simulink model "control"  (R2020b)
settings: Solver=VariableStepAuto  StartTime=0.0  StopTime=10.0  RelTol=1e-3
settings Model: Creator=Varun  LastModifiedBy=Varun
settings DataIOCC: SaveOutput=off  SaveTime=off

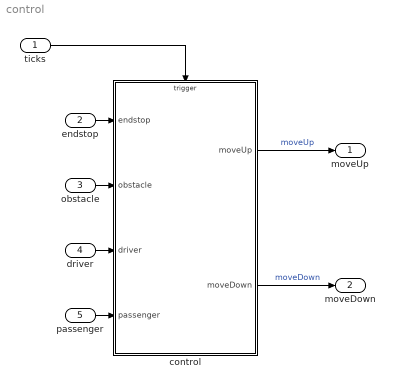
== system control ==
  ticks : Inport  OutDataTypeStr=double  PortDimensions=1
  endstop : Inport  Port=2  OutDataTypeStr=boolean  PortDimensions=1
  obstacle : Inport  Port=3  OutDataTypeStr=boolean  PortDimensions=1
  driver : Inport  Port=4  OutDataTypeStr=boolean  PortDimensions=3
  passenger : Inport  Port=5  OutDataTypeStr=boolean  PortDimensions=3
  control : Stateflow chart  TreatAsAtomicUnit=on
  moveUp : Outport  OutDataTypeStr=boolean  PortDimensions=1
  moveDown : Outport  Port=2  OutDataTypeStr=boolean  PortDimensions=1
  wires:
  passenger/1 -> control/4(passenger)
  obstacle/1 -> control/2(obstacle)
  control/2(moveDown) -> moveDown/1  "moveDown"
  ticks/1 -> control/Trigger
  control/1(moveUp) -> moveUp/1  "moveUp"
  endstop/1 -> control/1(endstop)
  driver/1 -> control/3(driver)

== stateflow chart control/control ==
  settings: executeAtInitialization=1
  state safe
    state driverNeutral
      entry:
      moveUp = 0;
      moveDown = 0;
      state passengerneutral
        entry:
        moveUp = 0;
        moveDown = 0;
      state passengerDown
        entry: moveDown = 1;
        exit: moveDown = 0;
        state iniPassengerDown
        state passengerDown
        state autoPassengerDown
        iniPassengerDown -> (junction 54) : after(100,ticks)
        (junction 54) -> autoPassengerDown [order 1] : [passenger[1]]
        (junction 54) -> safe.driverNeutral.passengerDown.passengerDown [order 2]
      state passengerUp
        entry: moveUp = 1;
        exit: moveUp = 0;
        state iniPassengerUp
        state PassengerUp
        state autoPassengerUp
        iniPassengerUp -> (junction 55) : after(100,ticks)
        (junction 55) -> PassengerUp [order 2]
        (junction 55) -> autoPassengerUp [order 1] : [passenger[1]]
      (default) -> passengerneutral
      passengerneutral -> iniPassengerUp [order 1] : [passenger[2]]
      passengerneutral -> iniPassengerDown [order 2] : [passenger[3]]
      safe.driverNeutral.passengerDown.passengerDown -> passengerneutral : [passenger[1]]
      safe.driverNeutral.passengerDown -> passengerneutral [order 1] : [endstop]
      PassengerUp -> passengerneutral : [passenger[1]]
      passengerUp -> passengerneutral [order 2] : [endstop]
      safe.driverNeutral.passengerDown -> PassengerUp [order 2] : [passenger[2]]
      passengerUp -> safe.driverNeutral.passengerDown.passengerDown [order 1] : [passenger[3]]
    state driverDown
      entry: moveDown = 1;
      exit: moveDown = 0;
      state iniDriverDown
      state autoDriverDown
      state DriverDown
      iniDriverDown -> (junction 56) : after(100,ticks)
      (junction 56) -> autoDriverDown [order 1] : [driver[1]]
      (junction 56) -> DriverDown [order 2]
    state driverUp
      entry: moveUp = 1;
      exit: moveUp = 0;
      state iniDriverUp
      state DriverUp
      state autoDriverUp
      iniDriverUp -> (junction 57) : after(100,ticks)
      (junction 57) -> DriverUp [order 2]
      (junction 57) -> autoDriverUp [order 1] : [driver[1]]
    (default) -> driverNeutral
    driverNeutral -> iniDriverDown [order 2] : [driver[3]]
    DriverDown -> driverNeutral : [driver[1]]
    driverDown -> driverNeutral [order 1] : [endstop]
    DriverUp -> driverNeutral : [driver[1]]
    driverUp -> driverNeutral [order 2] : [endstop]
    driverNeutral -> iniDriverUp [order 1] : [driver[2]]
    driverDown -> DriverUp [order 2] : [driver[2]]
    driverUp -> DriverDown [order 1] : [driver[3]]
  state emergencyDown
    entry:
    moveUp = 0;
    moveDown = 1;
  emergencyDown -> passengerneutral : [endstop | after(100,ticks)]
  (default) -> safe
  safe -> emergencyDown : [obstacle]
  data: moveUp output boolean; moveDown output boolean; endstop input boolean; obstacle input boolean; driver input boolean size=3; passenger input boolean size=3
  events: ticks input EITHER_EDGE_EVENT
